simulink model "control2_irb"  (R2019a)
settings: Solver=ode3  StartTime=0.0  StopTime=22  FixedStep=0.004  RelTol=1e-3  EnableMultiTasking=on
values from neighbouring files (symbols this model uses):
  a_max = [50 50 50 50]    [RUN.m]
  K_0 = [  5         0         0         0 ... (first row only)    [RUN.m]    (also in fitt.m = [  E         0         0         0)
  K_1 = [5.0000         0         0         0 ... (first row only)    [RUN.m]    (also in fitt.m = [a         0         0         0)
  Q_A = Robo.ikine(T_A,'mask',[1, 1, 1, 0, 0 ,0], 'verbose')    [IRB_trajectory2.m]    (also in RUN.m = [0.0951    0.1937    0.0007         0])
  torque_max = [300 150 150 28]    [RUN.m]
settings Model: Creator=Valdir Jr  LastModifiedBy=Valdir Jr

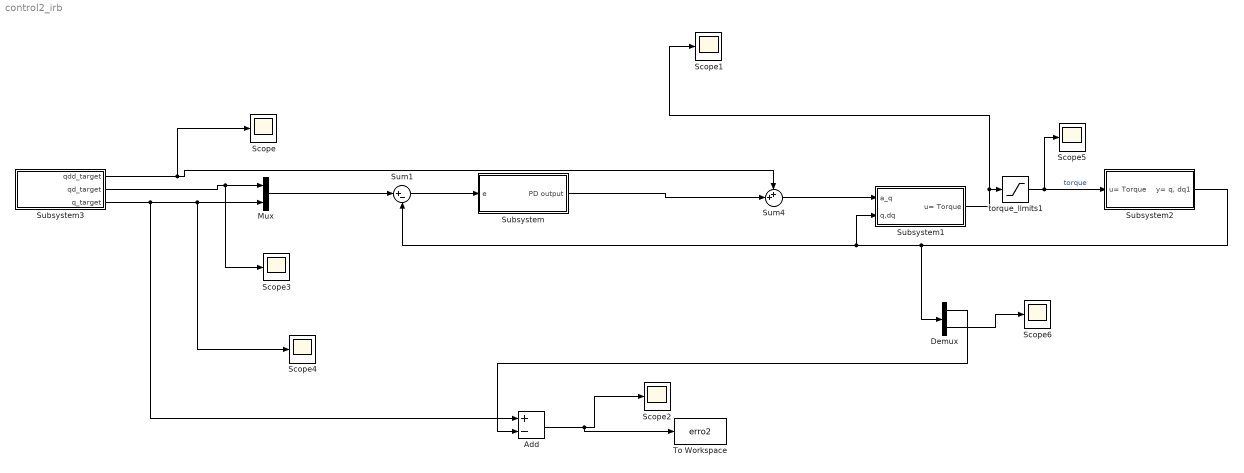
== system control2_irb ==
  Add : Sum  Inputs=+-
  Demux : Demux  Outputs=2
  Mux : Mux  Inputs=2
  Scope{,1..6} (7 alike) : Scope
  Subsystem : Subsystem
  Subsystem1 : Subsystem
  Subsystem2 : Subsystem
  Subsystem3 : Subsystem
  Sum1 : Sum  Inputs=|+-
  Sum4 : Sum  Inputs=++|
  To Workspace : ToWorkspace  VariableName=erro2  SaveFormat=Timeseries  SampleTime=-1
  torque_limits1 : Saturate  UpperLimit=torque_max  LowerLimit=-torque_max
  wires:
  Subsystem3/1(qdd_target) -> Sum4/1, Scope/1
  Subsystem3/2(qd_target) -> Scope3/1, Mux/1
  Subsystem3/3(q_target) -> Add/1, Scope4/1, Mux/2
  Mux/1 -> Sum1/1
  Sum1/1 -> Subsystem/1(e)
  Sum4/1 -> Subsystem1/1(a_q)
  Subsystem1/1(u= Torque) -> Scope1/1, torque_limits1/1
  Subsystem2/1("y= q, dq1") -> Demux/1, Subsystem1/2(q,dq), Sum1/2
  torque_limits1/1 -> Subsystem2/1(u= Torque), Scope5/1  "torque"
  Add/1 -> To Workspace/1, Scope2/1
  Demux/1 -> Add/2
  Subsystem/1(PD output) -> Sum4/2
  Demux/2 -> Scope6/1

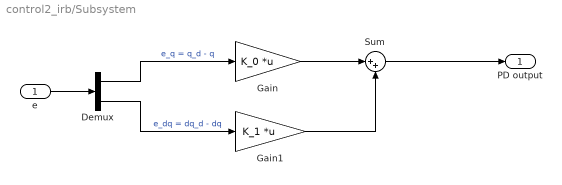
== system control2_irb/Subsystem ==
  e : Inport
  Demux : Demux  Outputs=[4 4]
  Gain : Gain  Gain=K_0  Multiplication=Matrix(K*u) (u vector)
  Gain1 : Gain  Gain=K_1  Multiplication=Matrix(K*u) (u vector)
  Sum : Sum  Inputs=|++
  PD output : Outport
  wires:
  Demux/2 -> Gain1/1  "e_dq = dq_d - dq"
  Demux/1 -> Gain/1  "e_q = q_d - q"
  Gain/1 -> Sum/1
  Gain1/1 -> Sum/2
  Sum/1 -> PD output/1
  e/1 -> Demux/1

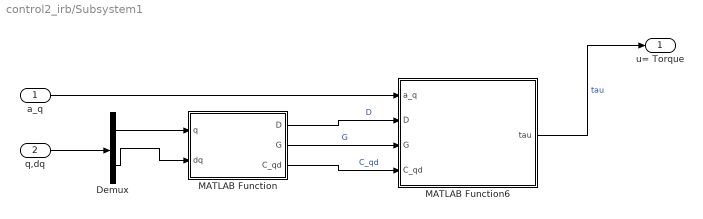
== system control2_irb/Subsystem1 ==
  a_q : Inport
  q,dq : Inport  Port=2
  Demux : Demux  Outputs=[4 4]
  MATLAB Function : MATLAB Function  TreatAsAtomicUnit=on
  MATLAB Function6 : MATLAB Function  TreatAsAtomicUnit=on
  u= Torque : Outport
  wires:
  MATLAB Function6/1(tau) -> u= Torque/1  "tau"
  Demux/2 -> MATLAB Function/2(dq)
  MATLAB Function/1(D) -> MATLAB Function6/2(D)  "D"
  q,dq/1 -> Demux/1
  Demux/1 -> MATLAB Function/1(q)
  MATLAB Function/2(G) -> MATLAB Function6/3(G)  "G"
  MATLAB Function/3(C_qd) -> MATLAB Function6/4(C_qd)  "C_qd"
  a_q/1 -> MATLAB Function6/1(a_q)

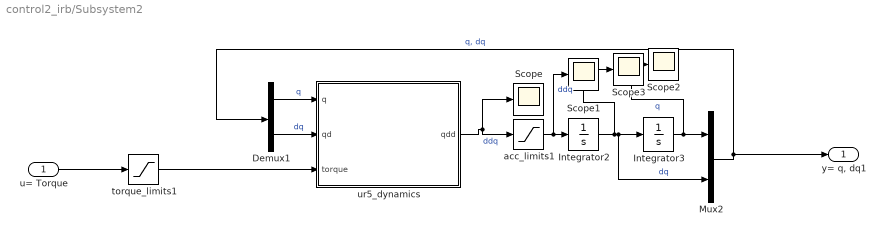
== system control2_irb/Subsystem2 ==
  u= Torque : Inport
  Demux1 : Demux  Outputs=[4 4]
  Integrator2 : Integrator  InitialCondition=Q_A  LimitOutput=on  UpperSaturationLimit="[3.4000    3.4000    15    3.4000]"  LowerSaturationLimit="-[3.4000    3.4000    15    3.4000]"  ContinuousStateAttributes='velocity'
  Integrator3 : Integrator  InitialCondition=Q_A  LimitOutput=on  UpperSaturationLimit="[6.2832    6.2832    6.2832    6.2832]"  LowerSaturationLimit="-[6.2832    6.2832    6.2832    6.2832]"  ContinuousStateAttributes='position'
  Mux2 : Mux  Inputs=[4 4]
  Scope{,1..3} (4 alike) : Scope
  acc_limits1 : Saturate  UpperLimit=a_max  LowerLimit=-a_max
  torque_limits1 : Saturate  UpperLimit="[150   150   150   28]"  LowerLimit="-[150   150   150   28]"
  ur5_dynamics : MATLAB Function  TreatAsAtomicUnit=on
  "y= q, dq1" : Outport
  wires:
  Demux1/1 -> ur5_dynamics/1(q)  "q"
  Integrator2/1 -> Scope3/1, Integrator3/1, Mux2/2  "dq"
  ur5_dynamics/1(qdd) -> acc_limits1/1, Scope/1  "ddq"
  Mux2/1 -> "y= q, dq1"/1, Demux1/1  "q, dq"
  acc_limits1/1 -> Scope1/1, Integrator2/1  "ddq"
  torque_limits1/1 -> ur5_dynamics/3(torque)
  Demux1/2 -> ur5_dynamics/2(qd)  "dq"
  Integrator3/1 -> Scope2/1, Mux2/1  "q"
  u= Torque/1 -> torque_limits1/1

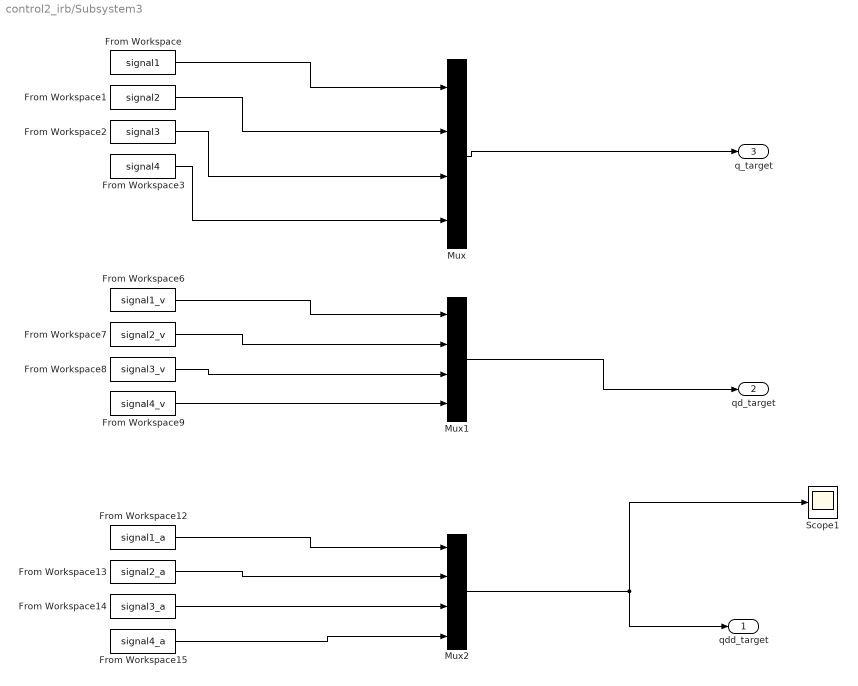
== system control2_irb/Subsystem3 ==
  From Workspace : FromWorkspace  VariableName=signal1  SampleTime=0
  From Workspace1 : FromWorkspace  VariableName=signal2  SampleTime=0
  From Workspace12 : FromWorkspace  VariableName=signal1_a  SampleTime=0
  From Workspace13 : FromWorkspace  VariableName=signal2_a  SampleTime=0
  From Workspace14 : FromWorkspace  VariableName=signal3_a  SampleTime=0
  From Workspace15 : FromWorkspace  VariableName=signal4_a  SampleTime=0
  From Workspace2 : FromWorkspace  VariableName=signal3  SampleTime=0
  From Workspace3 : FromWorkspace  VariableName=signal4  SampleTime=0
  From Workspace6 : FromWorkspace  VariableName=signal1_v  SampleTime=0
  From Workspace7 : FromWorkspace  VariableName=signal2_v  SampleTime=0
  From Workspace8 : FromWorkspace  VariableName=signal3_v  SampleTime=0
  From Workspace9 : FromWorkspace  VariableName=signal4_v  SampleTime=0
  Mux : Mux
  Mux1 : Mux
  Mux2 : Mux
  Scope1 : Scope
  qdd_target : Outport
  qd_target : Outport  Port=2
  q_target : Outport  Port=3
  wires:
  Mux/1 -> q_target/1
  Mux1/1 -> qd_target/1
  Mux2/1 -> qdd_target/1, Scope1/1
  From Workspace/1 -> Mux/1
  From Workspace1/1 -> Mux/2
  From Workspace2/1 -> Mux/3
  From Workspace3/1 -> Mux/4
  From Workspace6/1 -> Mux1/1
  From Workspace7/1 -> Mux1/2
  From Workspace8/1 -> Mux1/3
  From Workspace9/1 -> Mux1/4
  From Workspace12/1 -> Mux2/1
  From Workspace13/1 -> Mux2/2
  From Workspace14/1 -> Mux2/3
  From Workspace15/1 -> Mux2/4

== matlab function control2_irb/Subsystem1/MATLAB Function ==
  data: q input; D output; dq input; G output; C_qd output
function [ D, G, C_qd ] = IRB_Matrices( q, dq)
[ D, G, C_qd ] = IRB_getMatrices( q, dq );

== matlab function control2_irb/Subsystem2/ur5_dynamics ==
  data: q input; qd input; torque input; qdd output
function qdd = IRB_dynamics( q, qd, torque )
%#codegen
%Returns the acceleration of the manipulator based on its dynamics
[ D, G, CDq ] = IRB_getMatrices( q, qd );

qdd = D \ (torque - CDq - G);

== matlab function control2_irb/Subsystem1/MATLAB Function6 ==
  data: a_q input; D input; G input; C_qd input; tau output
function tau = IRB_invDynamics(a_q, D, G, C_qd)

tau = D*a_q + C_qd + G;
